simulink model "simulation_solution"  (R2019b)
settings: Solver=FixedStepAuto  StartTime=0.0  StopTime=simulation_duration  FixedStep=simulation_step  RelTol=1e-3
values from neighbouring files (symbols this model uses):
  angular_speed_max = deg2rad(45)    [init.m]
  dead_zone = 0.6    [init.m]
  init_angle = 0    [init.m]
  init_position = [0; 0]    [init.m]
  map_bounds = 10    [init.m]
  simulation_step = 0.1    [init.m]
  speed_max = 5    [init.m]
  x_ref_frequency = 0.025    [init.m]
  x_ref_mag = 7    [init.m]
  y_ref_frequency = 0.05    [init.m]
  y_ref_mag = 3    [init.m]
  y_ref_phase = 0    [init.m]
settings Model: Creator=grousseau  LastModifiedBy=grousseau

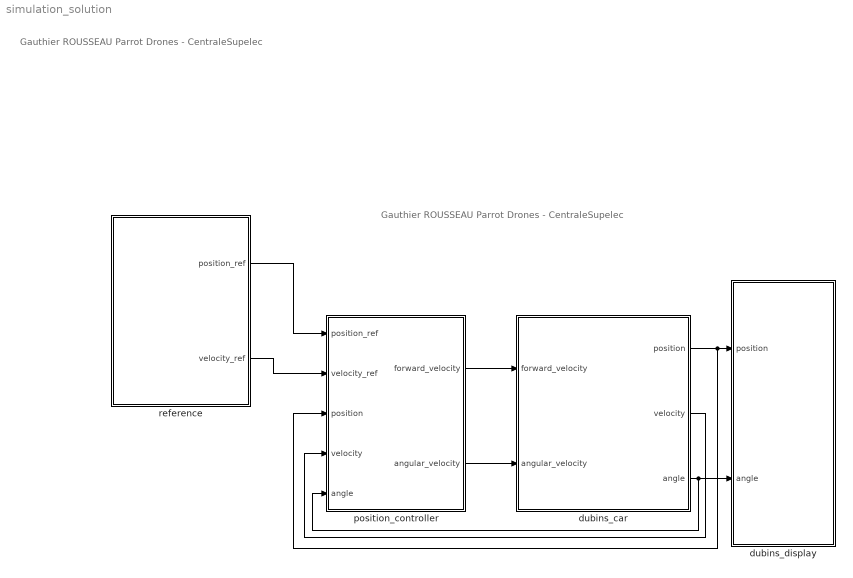
== system simulation_solution ==
  note: Gauthier ROUSSEAU
      | Parrot Drones - CentraleSupelec
  note: Gauthier ROUSSEAU
      | Parrot Drones - CentraleSupelec
  dubins_car : Subsystem
  dubins_display : Subsystem
  position_controller : Subsystem
  reference : Subsystem
  wires:
  dubins_car/1(position) -> position_controller/3(position), dubins_display/1(position)
  dubins_car/3(angle) -> dubins_display/2(angle), position_controller/5(angle)
  position_controller/1(forward_velocity) -> dubins_car/1(forward_velocity)
  position_controller/2(angular_velocity) -> dubins_car/2(angular_velocity)
  dubins_car/2(velocity) -> position_controller/4(velocity)
  reference/2(velocity_ref) -> position_controller/2(velocity_ref)
  reference/1(position_ref) -> position_controller/1(position_ref)

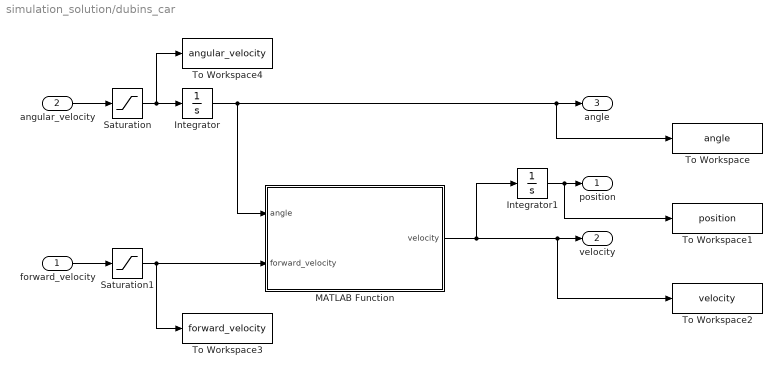
== system simulation_solution/dubins_car ==
  forward_velocity : Inport
  angular_velocity : Inport  Port=2
  Integrator : Integrator  InitialCondition=init_angle
  Integrator1 : Integrator  InitialCondition=init_position
  MATLAB Function : MATLAB Function  TreatAsAtomicUnit=on
  Saturation : Saturate  UpperLimit=angular_speed_max  LowerLimit=-angular_speed_max
  Saturation1 : Saturate  UpperLimit=speed_max  LowerLimit=-speed_max
  To Workspace : ToWorkspace  VariableName=angle  SaveFormat=Timeseries  SampleTime=-1
  To Workspace1 : ToWorkspace  VariableName=position  SaveFormat=Timeseries  SampleTime=-1
  To Workspace2 : ToWorkspace  VariableName=velocity  SaveFormat=Timeseries  SampleTime=-1
  To Workspace3 : ToWorkspace  VariableName=forward_velocity  SaveFormat=Timeseries  SampleTime=-1
  To Workspace4 : ToWorkspace  VariableName=angular_velocity  SaveFormat=Timeseries  SampleTime=-1
  position : Outport
  velocity : Outport  Port=2
  angle : Outport  Port=3
  wires:
  Integrator/1 -> To Workspace/1, angle/1, MATLAB Function/1(angle)
  MATLAB Function/1(velocity) -> Integrator1/1, To Workspace2/1, velocity/1
  Integrator1/1 -> To Workspace1/1, position/1
  Saturation/1 -> To Workspace4/1, Integrator/1
  angular_velocity/1 -> Saturation/1
  forward_velocity/1 -> Saturation1/1
  Saturation1/1 -> To Workspace3/1, MATLAB Function/2(forward_velocity)

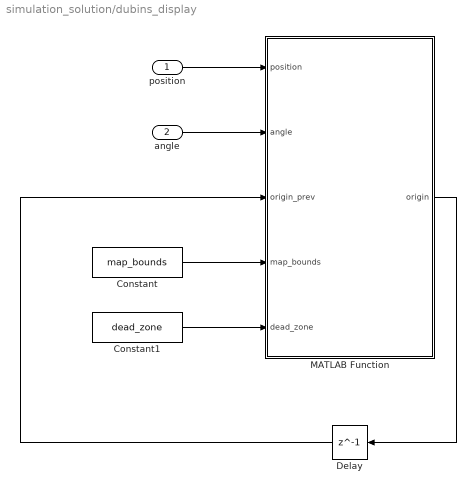
== system simulation_solution/dubins_display ==
  position : Inport
  angle : Inport  Port=2
  Constant : Constant  Value=map_bounds
  Constant1 : Constant  Value=dead_zone
  Delay : Delay  DelayLength=1  InitialCondition=init_position  SampleTime=simulation_step
  MATLAB Function : MATLAB Function  TreatAsAtomicUnit=on
  wires:
  position/1 -> MATLAB Function/1(position)
  angle/1 -> MATLAB Function/2(angle)
  Constant/1 -> MATLAB Function/4(map_bounds)
  Constant1/1 -> MATLAB Function/5(dead_zone)
  MATLAB Function/1(origin) -> Delay/1
  Delay/1 -> MATLAB Function/3(origin_prev)

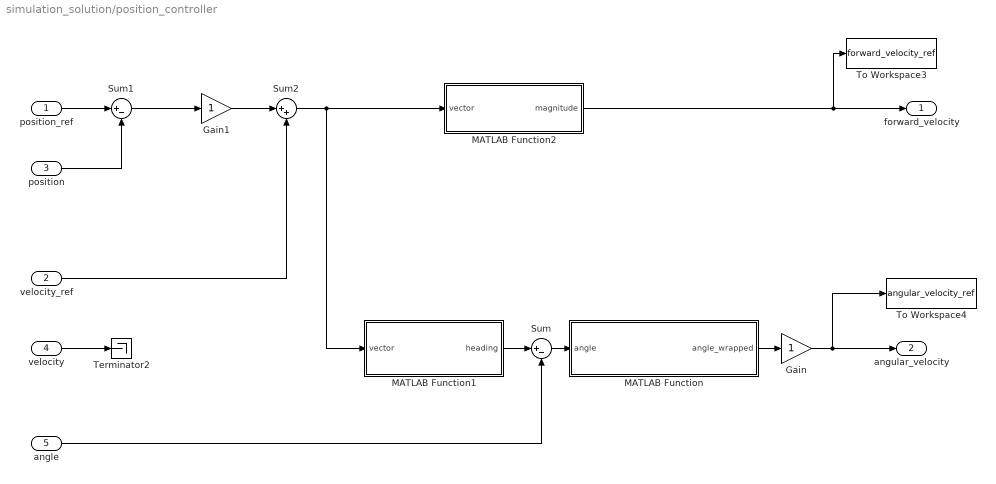
== system simulation_solution/position_controller ==
  position_ref : Inport
  velocity_ref : Inport  Port=2
  position : Inport  Port=3
  velocity : Inport  Port=4
  angle : Inport  Port=5
  Gain : Gain
  Gain1 : Gain
  MATLAB Function : MATLAB Function  TreatAsAtomicUnit=on
  MATLAB Function1 : MATLAB Function  TreatAsAtomicUnit=on
  MATLAB Function2 : MATLAB Function  TreatAsAtomicUnit=on
  Sum : Sum  Inputs=|+-
  Sum1 : Sum  Inputs=|+-
  Sum2 : Sum  Inputs=|++
  Terminator2 : Terminator
  To Workspace3 : ToWorkspace  VariableName=forward_velocity_ref  SaveFormat=Timeseries  SampleTime=-1
  To Workspace4 : ToWorkspace  VariableName=angular_velocity_ref  SaveFormat=Timeseries  SampleTime=-1
  forward_velocity : Outport
  angular_velocity : Outport  Port=2
  wires:
  position_ref/1 -> Sum1/1
  position/1 -> Sum1/2
  velocity/1 -> Terminator2/1
  Gain/1 -> To Workspace4/1, angular_velocity/1
  velocity_ref/1 -> Sum2/2
  angle/1 -> Sum/2
  MATLAB Function2/1(magnitude) -> To Workspace3/1, forward_velocity/1
  Sum/1 -> MATLAB Function/1(angle)
  MATLAB Function/1(angle_wrapped) -> Gain/1
  Sum1/1 -> Gain1/1
  Gain1/1 -> Sum2/1
  MATLAB Function1/1(heading) -> Sum/1
  Sum2/1 -> MATLAB Function2/1(vector), MATLAB Function1/1(vector)

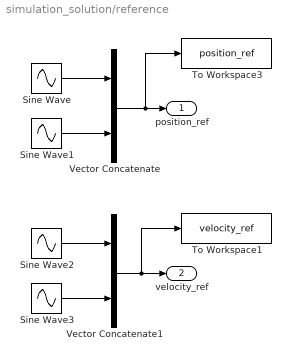
== system simulation_solution/reference ==
  Sine Wave : Sin  Amplitude=x_ref_mag  Frequency=x_ref_frequency * (2*pi)  SampleTime=0
  Sine Wave1 : Sin  Amplitude=y_ref_mag  Frequency=y_ref_frequency * (2*pi)  Phase=y_ref_phase  SampleTime=0
  Sine Wave2 : Sin  Amplitude=x_ref_mag * x_ref_frequency * (2*pi)  Frequency=x_ref_frequency * (2*pi)  Phase=pi/2  SampleTime=0
  Sine Wave3 : Sin  Amplitude=y_ref_mag * y_ref_frequency * (2*pi)  Frequency=y_ref_frequency * (2*pi)  Phase=y_ref_phase + pi/2  SampleTime=0
  To Workspace1 : ToWorkspace  VariableName=velocity_ref  SaveFormat=Timeseries  SampleTime=-1
  To Workspace3 : ToWorkspace  VariableName=position_ref  SaveFormat=Timeseries  SampleTime=-1
  Vector Concatenate : Concatenate
  Vector Concatenate1 : Concatenate
  position_ref : Outport
  velocity_ref : Outport  Port=2
  wires:
  Sine Wave1/1 -> Vector Concatenate/2
  Sine Wave/1 -> Vector Concatenate/1
  Sine Wave2/1 -> Vector Concatenate1/1
  Sine Wave3/1 -> Vector Concatenate1/2
  Vector Concatenate1/1 -> To Workspace1/1, velocity_ref/1
  Vector Concatenate/1 -> To Workspace3/1, position_ref/1

== matlab function simulation_solution/dubins_display/MATLAB Function ==
  data: position input; angle input; origin_prev input; map_bounds input; dead_zone input; origin output
function origin = display_dubins(position, angle, origin_prev, map_bounds, dead_zone)

x_car = [0.7 -1  -1    0.7 1.3 0.7 -1   -1    0.7 0.7];
y_car = [0.7 0.7 -0.7 -0.7 0   0.7 -0.7  0.7 -0.7 0.7];

c = cos(angle); s = sin(angle);
x_draw = c * x_car - s * y_car;
y_draw = s * x_car + c * y_car;

x_draw = x_draw + position(1);
y_draw = y_draw + position(2);

dead_zone_start = dead_zone * map_bounds;
delta = position - origin_prev;
if abs(delta(1)) > dead_zone_start
    ratio = dead_zone_start / abs(delta(1));
    delta = ratio * delta;
end
if abs(delta(2)) > dead_zone_start
    ratio = dead_zone_start / abs(delta(2));
    delta = ratio * delta;
end
origin = position - delta;

% figure(2);
plot(x_draw, y_draw, 'r', 'linewidth', 1.5);
grid on;
xlim([-map_bounds map_bounds]+origin(1));
ylim([-map_bounds map_bounds]+origin(2));
daspect([1 1 1]);

drawnow;
end

== matlab function simulation_solution/dubins_car/MATLAB Function ==
  data: angle input; velocity output; forward_velocity input
function velocity = dubin_model(angle, forward_velocity)

velocity = [forward_velocity * cos(angle)
            forward_velocity * sin(angle)];
end

== matlab function simulation_solution/position_controller/MATLAB Function ==
  data: angle input; angle_wrapped output
function angle_wrapped = wrap_to_pi(angle)
angle_wrapped = mod(angle, 2*pi);

if angle_wrapped > pi
    angle_wrapped = angle_wrapped - 2*pi;
end
end

== matlab function simulation_solution/position_controller/MATLAB Function1 ==
  data: vector input; heading output
function heading = vector_direction(vector)
heading = atan2(vector(2), vector(1));
end

== matlab function simulation_solution/position_controller/MATLAB Function2 ==
  data: vector input; magnitude output
function magnitude = norm_2(vector)
magnitude = norm(vector);
end
